simulink model "eightenPulseRectifier"  (R2024a)
settings: Solver=VariableStepAuto  StartTime=0.0  StopTime=.2  MaxStep=.0001  RelTol=1e-3
libraries: spsThyristorLib x60, spsVoltageMeasurementLib x47, spsControlledVoltageSourceLib x15, spsSeriesRLCBranchLib x9, spsZigzagPhaseShiftingTransformerLib x8, spsGroundLib x6, spsThreePhaseTransformerTwoWindingsLib x4, spsMeanLib x3, spsUniversalBridgeLib x3, slpidlib x1, simulink_extras x1, sps_lib x1
(part 1 of 2)
settings Model: Creator=User  LastModifiedBy=Admin

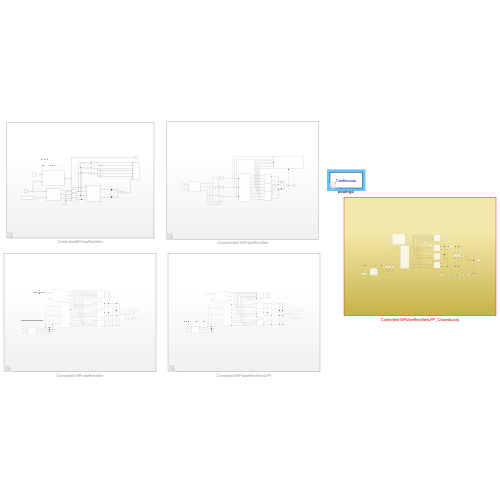
[thumbnail: Simulink's stored preview of the top-level diagram]
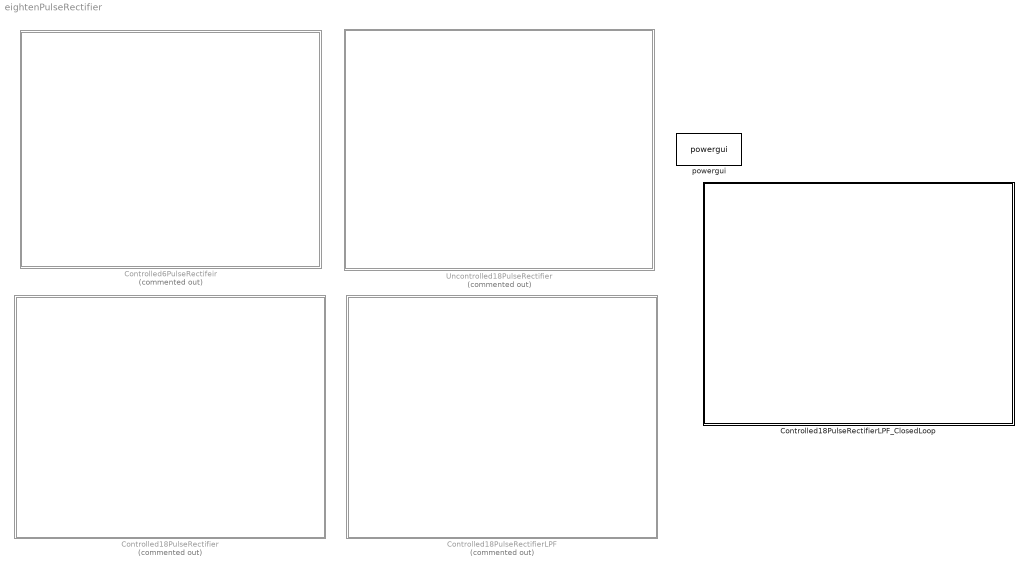
== system eightenPulseRectifier ==
  Controlled18PulseRectifier : Subsystem  Commented=on
  Controlled18PulseRectifierLPF : Subsystem  Commented=on
  Controlled18PulseRectifierLPF_ClosedLoop : Subsystem
  Controlled6PulseRectifeir : Subsystem  Commented=on
  Uncontrolled18PulseRectifier : Subsystem  Commented=on
  powergui : sps_lib/powergui  Priority=1  SimulationMode=Continuous  SampleTime=50e-6  frequency=60  Iterations=50  frequencyindice=0  Pbase=100e6  ErrMax=1e-4  UnitsV=kV  UnitsW=MW  buscounter=0  FunctionMessages=off  echomessages=off  EnableUseOfTLC=off  CurrentSourceSwitches=off  DisableSnubberDevices=off  DisableRonSwitches=off  DisableVfSwitches=off  DisplayEquations=off  AutomaticDiscreteSolvers=off  SolverType=Tustin/Backward Euler (TBE)  Interpol=off  ExternalGateDelay=off  methode=off  Ts=100  x0status=blocks  SPID=on  SwTol=0  HookPort=off  NonlinearTolerance=1e-4  nMaxIteration=100  ContinueOnMaxIteration=off  RestoreLinks=warning  ResistiveCurrentMeasurement=off  Frange=[0:2:500]  Ylog=off  Xlog=on  ShowGrid=off  save=off  variable=ZData  structure=0  ZoomFFT=off  StartTime=0.0  cycles=1  DisplayStyle=1  fundamental=60  FreqAxis=off  MaxFrequency=1000  frequencyindicesteady=1  RmsSteady=1  display=off

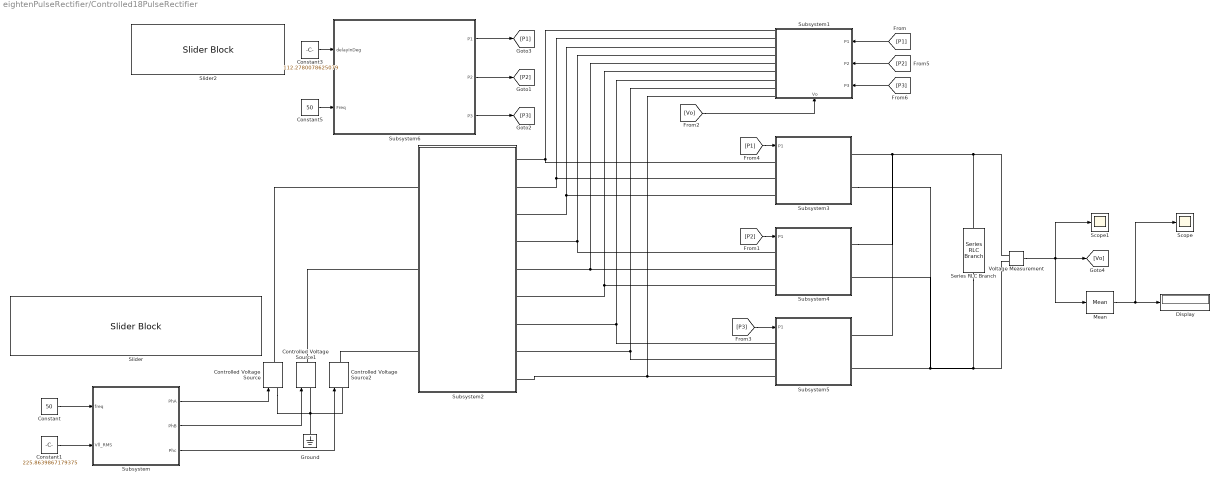
== system eightenPulseRectifier/Controlled18PulseRectifier ==
  Constant : Constant  Value=50
  Constant1 : Constant  Value=225.8639867179375
  Constant3 : Constant  Value=112.2780078625079
  Constant5 : Constant  Value=50
  Controlled Voltage Source : spsControlledVoltageSourceLib/Controlled Voltage Source  Initialize=on  Source_Type=AC  Amplitude=0  Phase=0  Frequency=0  Measurements=None
  Controlled Voltage Source1 : spsControlledVoltageSourceLib/Controlled Voltage Source  Initialize=on  Source_Type=AC  Amplitude=0  Phase=0  Frequency=0  Measurements=None
  Controlled Voltage Source2 : spsControlledVoltageSourceLib/Controlled Voltage Source  Initialize=on  Source_Type=AC  Amplitude=0  Phase=0  Frequency=0  Measurements=None
  Display : Display
  Ground : spsGroundLib/Ground  LConnTagsString=a
  Mean : spsMeanLib/Mean  Freq=60  Vinit=0  Ts=0
  Scope : Scope
  Scope1 : Scope
  Series RLC Branch : spsSeriesRLCBranchLib/Series RLC Branch  LConnTagsString=__new0  RConnTagsString=__new0  BranchType=R  Resistance=1.45  Inductance=1e-3  SetiL0=off  InitialCurrent=0  Capacitance=1e-6  Setx0=off  InitialVoltage=0  Measurements=None
  Slider : SliderBlock  ScaleMin=187  ScaleMax=253
  Slider2 : SliderBlock  ScaleMin=50  ScaleMax=180
  Subsystem : Subsystem
  Subsystem1 : Subsystem
      settings: PortSchema="{\"entries\":[{\"content\":{\"sides\":[{\"content\":{\"connectorIds\":[\"LConn1\",\"LConn2\",\"LConn3\",\"LConn4\",\"LConn5\",\"LConn6\",\"LConn7\",\"LConn8\",\"LConn9\"]},\"type\":\"ConnectorPlacement.EquallySpacedRectSide\",\"uuid\":\"c528b960-0f89-4916-bc59-feafc106a6fa\"},{\"content\":{\"connectorIds\":[\"In2\",\"In3\",\"In4\"],\"side\":\"RIGHT\"},\"type\":\"ConnectorPlacement.EquallySpacedRectSide\",\"uuid\":\"71a864a5-f7f4-48a7-95f9-d8a7d95b84d2\"},{\"content\":{\"side\":\"TOP\"},\"type\":\"ConnectorPlacement.EquallySpacedRectSide\",\"uuid\":\"57c5c08c-8233-4b40-a9fb-e09e67286da5\"},{\"content\":{\"connectorIds\":[\"In1\"],\"side\":\"BOTTOM\"},\"type\":\"ConnectorPlacement.EquallySpacedRectSide\",\"uuid\":\"030adcd8-0531-402c-81c9-62e294f4d5af\"}]},\"type\":\"ConnectorPlacement.EquallySpacedConnector\",\"uuid\":\"216ad3eb-0ca6-4d39-b862-04814928268f\"}],\"packageUris\":[\"http://schema.mathworks.com/mf0/Connector/R2020b\"],\"version\":\"1.0\"}"
  Subsystem2 : Subsystem
  Subsystem3 : Subsystem
  Subsystem4 : Subsystem
  Subsystem5 : Subsystem
  Subsystem6 : Subsystem
  Voltage Measurement : spsVoltageMeasurementLib/Voltage Measurement  PhasorSimulation=off  OutputType=Complex  PSBequivalent=0
  wires:
  Constant/1 -> Subsystem/1(freq)
  Constant1/1 -> Subsystem/2(Vll_RMS)
  Subsystem/3(Phc) -> Controlled Voltage Source2/1
  Subsystem/2(PhB) -> Controlled Voltage Source1/1
  Subsystem/1(PhA) -> Controlled Voltage Source/1
  [P3] -> Subsystem5/1(P1)
  Subsystem6/2(P2) -> [P2]
  Subsystem6/3(P3) -> [P3]
  Voltage Measurement/1 -> Mean/1, [Vo], Scope1/1
  [Vo] -> Subsystem1/1(Vo)
  [P1] -> Subsystem3/1(P1)
  [P2] -> Subsystem4/1(P1)
  Subsystem6/1(P1) -> [P1]
  [P1] -> Subsystem1/2(P1)
  [P2] -> Subsystem1/3(P2)
  [P3] -> Subsystem1/4(P3)
  Constant5/1 -> Subsystem6/2(Freq)
  Constant3/1 -> Subsystem6/1(delayInDeg)
  Mean/1 -> Scope/1, Display/1
  connections:
  Subsystem1/LConn9 -- Subsystem2/RConn9 -- Subsystem5/LConn3
  Subsystem1/LConn6 -- Subsystem4/LConn3 -- Subsystem2/RConn6
  Controlled Voltage Source/RConn1 -- Subsystem2/LConn1
  Subsystem1/LConn5 -- Subsystem2/RConn5 -- Subsystem4/LConn2
  Subsystem1/LConn7 -- Subsystem5/LConn1 -- Subsystem2/RConn7
  Subsystem1/LConn3 -- Subsystem2/RConn3 -- Subsystem3/LConn3
  Ground/LConn1 -- Controlled Voltage Source/LConn1 -- Controlled Voltage Source1/LConn1 -- Controlled Voltage Source2/LConn1
  Subsystem3/LConn2 -- Subsystem1/LConn2 -- Subsystem2/RConn2
  Voltage Measurement/LConn1 -- Subsystem4/RConn1 -- Subsystem5/RConn1 -- Subsystem3/RConn1 -- Series RLC Branch/LConn1
  Series RLC Branch/RConn1 -- Subsystem3/RConn2 -- Subsystem4/RConn2 -- Subsystem5/RConn2 -- Voltage Measurement/LConn2
  Subsystem1/LConn8 -- Subsystem5/LConn2 -- Subsystem2/RConn8
  Subsystem1/LConn4 -- Subsystem4/LConn1 -- Subsystem2/RConn4
  Controlled Voltage Source2/RConn1 -- Subsystem2/LConn3
  Controlled Voltage Source1/RConn1 -- Subsystem2/LConn2
  Subsystem1/LConn1 -- Subsystem3/LConn1 -- Subsystem2/RConn1

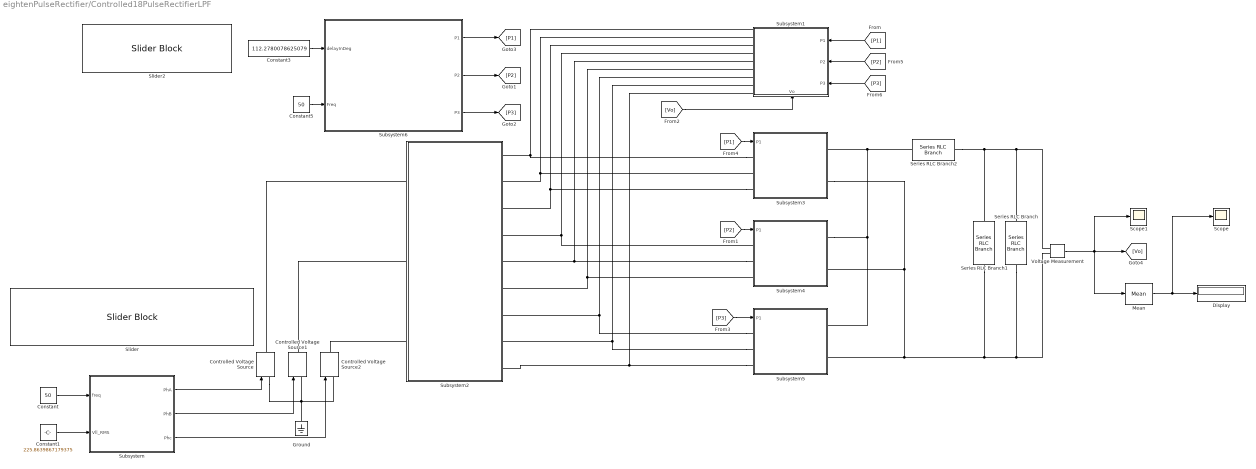
== system eightenPulseRectifier/Controlled18PulseRectifierLPF ==
  Constant : Constant  Value=50
  Constant1 : Constant  Value=225.8639867179375
  Constant3 : Constant  Value=112.2780078625079
  Constant5 : Constant  Value=50
  Controlled Voltage Source : spsControlledVoltageSourceLib/Controlled Voltage Source  Initialize=on  Source_Type=AC  Amplitude=0  Phase=0  Frequency=0  Measurements=None
  Controlled Voltage Source1 : spsControlledVoltageSourceLib/Controlled Voltage Source  Initialize=on  Source_Type=AC  Amplitude=0  Phase=0  Frequency=0  Measurements=None
  Controlled Voltage Source2 : spsControlledVoltageSourceLib/Controlled Voltage Source  Initialize=on  Source_Type=AC  Amplitude=0  Phase=0  Frequency=0  Measurements=None
  Display : Display
  Ground : spsGroundLib/Ground  LConnTagsString=a
  Mean : spsMeanLib/Mean  Freq=60  Vinit=0  Ts=0
  Scope : Scope
  Scope1 : Scope
  Series RLC Branch : spsSeriesRLCBranchLib/Series RLC Branch  LConnTagsString=__new0  RConnTagsString=__new0  BranchType=R  Resistance=1.45  Inductance=1e-3  SetiL0=off  InitialCurrent=0  Capacitance=1e-6  Setx0=off  InitialVoltage=0  Measurements=None
  Series RLC Branch1 : spsSeriesRLCBranchLib/Series RLC Branch  LConnTagsString=__new0  RConnTagsString=__new0  BranchType=C  Resistance=1.45  Inductance=1e-3  SetiL0=off  InitialCurrent=0  Capacitance=1500e-6  Setx0=off  InitialVoltage=0  Measurements=None
  Series RLC Branch2 : spsSeriesRLCBranchLib/Series RLC Branch  LConnTagsString=__new0  RConnTagsString=__new0  BranchType=L  Resistance=1.45  Inductance=2e-3  SetiL0=off  InitialCurrent=0  Capacitance=1e-6  Setx0=off  InitialVoltage=0  Measurements=None
  Slider : SliderBlock  ScaleMin=187  ScaleMax=253
  Slider2 : SliderBlock  ScaleMin=50  ScaleMax=180
  Subsystem : Subsystem
  Subsystem1 : Subsystem
      settings: PortSchema="{\"entries\":[{\"content\":{\"sides\":[{\"content\":{\"connectorIds\":[\"LConn1\",\"LConn2\",\"LConn3\",\"LConn4\",\"LConn5\",\"LConn6\",\"LConn7\",\"LConn8\",\"LConn9\"]},\"type\":\"ConnectorPlacement.EquallySpacedRectSide\",\"uuid\":\"c528b960-0f89-4916-bc59-feafc106a6fa\"},{\"content\":{\"connectorIds\":[\"In2\",\"In3\",\"In4\"],\"side\":\"RIGHT\"},\"type\":\"ConnectorPlacement.EquallySpacedRectSide\",\"uuid\":\"71a864a5-f7f4-48a7-95f9-d8a7d95b84d2\"},{\"content\":{\"side\":\"TOP\"},\"type\":\"ConnectorPlacement.EquallySpacedRectSide\",\"uuid\":\"57c5c08c-8233-4b40-a9fb-e09e67286da5\"},{\"content\":{\"connectorIds\":[\"In1\"],\"side\":\"BOTTOM\"},\"type\":\"ConnectorPlacement.EquallySpacedRectSide\",\"uuid\":\"030adcd8-0531-402c-81c9-62e294f4d5af\"}]},\"type\":\"ConnectorPlacement.EquallySpacedConnector\",\"uuid\":\"216ad3eb-0ca6-4d39-b862-04814928268f\"}],\"packageUris\":[\"http://schema.mathworks.com/mf0/Connector/R2020b\"],\"version\":\"1.0\"}"
  Subsystem2 : Subsystem
  Subsystem3 : Subsystem
  Subsystem4 : Subsystem
  Subsystem5 : Subsystem
  Subsystem6 : Subsystem
  Voltage Measurement : spsVoltageMeasurementLib/Voltage Measurement  PhasorSimulation=off  OutputType=Complex  PSBequivalent=0
  wires:
  Mean/1 -> Display/1, Scope/1
  Constant3/1 -> Subsystem6/1(delayInDeg)
  Constant5/1 -> Subsystem6/2(Freq)
  [P3] -> Subsystem1/4(P3)
  [P2] -> Subsystem1/3(P2)
  [P1] -> Subsystem1/2(P1)
  Subsystem6/1(P1) -> [P1]
  [P2] -> Subsystem4/1(P1)
  [P1] -> Subsystem3/1(P1)
  [Vo] -> Subsystem1/1(Vo)
  Voltage Measurement/1 -> Scope1/1, [Vo], Mean/1
  Subsystem6/3(P3) -> [P3]
  Subsystem6/2(P2) -> [P2]
  [P3] -> Subsystem5/1(P1)
  Subsystem/1(PhA) -> Controlled Voltage Source/1
  Subsystem/2(PhB) -> Controlled Voltage Source1/1
  Subsystem/3(Phc) -> Controlled Voltage Source2/1
  Constant1/1 -> Subsystem/2(Vll_RMS)
  Constant/1 -> Subsystem/1(freq)
  connections:
  Subsystem3/LConn1 -- Subsystem2/RConn1 -- Subsystem1/LConn1
  Controlled Voltage Source1/RConn1 -- Subsystem2/LConn2
  Controlled Voltage Source2/RConn1 -- Subsystem2/LConn3
  Subsystem2/RConn4 -- Subsystem1/LConn4 -- Subsystem4/LConn1
  Subsystem5/LConn2 -- Subsystem2/RConn8 -- Subsystem1/LConn8
  Voltage Measurement/LConn2 -- Series RLC Branch1/RConn1 -- Subsystem5/RConn2 -- Subsystem3/RConn2 -- Subsystem4/RConn2 -- Series RLC Branch/RConn1
  Subsystem3/RConn1 -- Series RLC Branch2/LConn1 -- Subsystem5/RConn1 -- Subsystem4/RConn1
  Subsystem2/RConn2 -- Subsystem1/LConn2 -- Subsystem3/LConn2
  Controlled Voltage Source2/LConn1 -- Controlled Voltage Source1/LConn1 -- Controlled Voltage Source/LConn1 -- Ground/LConn1
  Subsystem3/LConn3 -- Subsystem2/RConn3 -- Subsystem1/LConn3
  Subsystem5/LConn1 -- Subsystem2/RConn7 -- Subsystem1/LConn7
  Subsystem4/LConn2 -- Subsystem2/RConn5 -- Subsystem1/LConn5
  Controlled Voltage Source/RConn1 -- Subsystem2/LConn1
  Subsystem2/RConn6 -- Subsystem4/LConn3 -- Subsystem1/LConn6
  Subsystem5/LConn3 -- Subsystem2/RConn9 -- Subsystem1/LConn9
  Series RLC Branch/LConn1 -- Series RLC Branch1/LConn1 -- Series RLC Branch2/RConn1 -- Voltage Measurement/LConn1

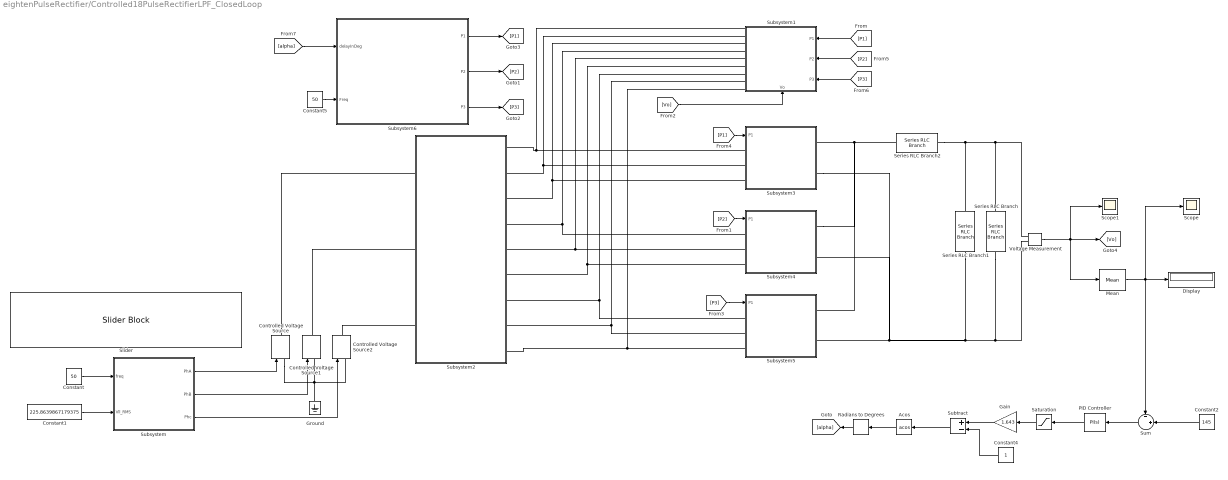
== system eightenPulseRectifier/Controlled18PulseRectifierLPF_ClosedLoop ==
  Acos : Trigonometry  Operator=acos
  Constant : Constant  Value=50
  Constant1 : Constant  Value=225.8639867179375
  Constant2 : Constant  Value=145
  Constant4 : Constant
  Constant5 : Constant  Value=50
  Controlled Voltage Source : spsControlledVoltageSourceLib/Controlled Voltage Source  Initialize=on  Source_Type=AC  Amplitude=0  Phase=0  Frequency=0  Measurements=None
  Controlled Voltage Source1 : spsControlledVoltageSourceLib/Controlled Voltage Source  Initialize=on  Source_Type=AC  Amplitude=0  Phase=0  Frequency=0  Measurements=None
  Controlled Voltage Source2 : spsControlledVoltageSourceLib/Controlled Voltage Source  Initialize=on  Source_Type=AC  Amplitude=0  Phase=0  Frequency=0  Measurements=None
  Display : Display
  Gain : Gain  Gain=1.643
  Ground : spsGroundLib/Ground  LConnTagsString=a
  Mean : spsMeanLib/Mean  Freq=60  Vinit=0  Ts=0
  PID Controller : slpidlib/PID Controller  Controller=PI  Form=Parallel  TimeDomain=Continuous-time  UseExternalTs=off  SampleTime=-1  IntegratorMethod=Forward Euler  FilterMethod=Forward Euler  ControllerParametersSource=internal  P=.02  I=5  UseKiTs=off  D=0  UseExternalDerivativeSource=off  N=100  UseFilter=on  TunerSelectOption=Transfer Function Based (PID Tuner App)  InitialConditionSource=internal  InitialConditionForIntegrator=0  InitialConditionForFilter=0  DifferentiatorICPrevScaledInput=0  ExternalReset=none  TrackingMode=off  Kt=1  LimitOutput=off  SatLimitsSource=internal  UpperSaturationLimit=.95  LowerSaturationLimit=.1  LinearizeAsGain=on  AntiWindupMode=clamping  Kb=1  LimitIntegrator=off  UpperIntegratorSaturationLimit=inf  LowerIntegratorSaturationLimit=-inf  POutMin=[]  POutMax=[]  IOutMin=[]  IOutMax=[]  DOutMin=[]  DOutMax=[]  NOutMin=[]  NOutMax=[]  SumOutMin=[]  SumOutMax=[]  SaturationOutMin=[]  SaturationOutMax=[]  PParamMin=[]  PParamMax=[]  IParamMin=[]  IParamMax=[]  DParamMin=[]  DParamMax=[]  NParamMin=[]  NParamMax=[]  KbParamMin=[]  KbParamMax=[]  KtParamMin=[]  KtParamMax=[]  KbOutMin=[]  KbOutMax=[]  KtOutMin=[]  KtOutMax=[]  IntegratorOutMin=[]  IntegratorOutMax=[]  FilterOutMin=[]  FilterOutMax=[]  SumI1OutMin=[]  SumI1OutMax=[]  SumI2OutMin=[]  SumI2OutMax=[]  SumI3OutMin=[]  SumI3OutMax=[]  SumI4OutMin=[]  SumI4OutMax=[]  SumDOutMin=[]  SumDOutMax=[]  DifferentiatorOutMin=[]  DifferentiatorOutMax=[]  FilterDiffOutCoefMin=[]  FilterDiffOutCoefMax=[]  ReciprocalOutMin=[]  ReciprocalOutMax=[]  SumDenOutMin=[]  SumDenOutMax=[]  SumNumOutMin=[]  SumNumOutMax=[]  DivideOutMin=[]  DivideOutMax=[]  UdiffTsProdOutMin=[]  UdiffTsProdOutMax=[]  NTsProdOutMin=[]  NTsProdOutMax=[]  UintegralTsProdOutMin=[]  UintegralTsProdOutMax=[]  UngainTsProdOutMin=[]  UngainTsProdOutMax=[]  ClampingZeroOutDataTypeStr=Inherit: Inherit via back propagation  ClampingZeroOutMin=[]  ClampingZeroOutMax=[]  FilterDenConstantOutDataTypeStr=Inherit: Inherit via back propagation  FilterDenConstantOutMin=[]  FilterDenConstantOutMax=[]  PCopyOutDataTypeStr=Inherit: Inherit via back propagation  PCopyOutMin=[]  PCopyOutMax=[]  NCopyOutDataTypeStr=Inherit: Inherit via back propagation  NCopyOutMin=[]  NCopyOutMax=[]  IntegratorContinuousStateAttributes=''  IntegratorStateMustResolveToSignalObject=off  IntegratorRTWStateStorageClass=Auto  FilterContinuousStateAttributes=''  FilterStateMustResolveToSignalObject=off  FilterRTWStateStorageClass=Auto  ParallelPVariant=InternalParameters  IdealPVariant=Disabled  IVariant=InternalParameters  DVariant=Disabled  IntegratorVariant=Continuous  SatVariant=Disabled  AWVariant=Passthrough  PCopyVariant=Disabled  TRVariant=Disabled  FdbkBlocksVariant=Forward  IdealPFdbkVariant=Disabled  SatFdbkVariant=Disabled  DerivativeFilterVariant=Disabled  NVariant=Disabled  NCopyVariant=Disabled_SignalSpec  FilterICVariant=Disabled  IntegratorICVariant=InternalICs  ExternalResetVariant=Disabled  TRSumVariant=Passthrough  SumFdbkVariant=Disabled  SumVariant=Sum_PI  TsampFilterVariant=InternalTs  TsampNgainVariant=Passthrough  TsampIntegralVariant=Disabled_SignalSpec  ExternalSaturationOutDataTypeStr=Inherit: Same as second input  DerivativeSourceVariant=Disabled
  Radians to Degrees : simulink_extras/Transformations/Radians to Degrees
  Saturation : Saturate  UpperLimit=.95  LowerLimit=.1
  Scope : Scope
  Scope1 : Scope
  Series RLC Branch : spsSeriesRLCBranchLib/Series RLC Branch  LConnTagsString=__new0  RConnTagsString=__new0  BranchType=R  Resistance=1.45  Inductance=1e-3  SetiL0=off  InitialCurrent=0  Capacitance=1e-6  Setx0=off  InitialVoltage=0  Measurements=None
  Series RLC Branch1 : spsSeriesRLCBranchLib/Series RLC Branch  LConnTagsString=__new0  RConnTagsString=__new0  BranchType=C  Resistance=1.45  Inductance=1e-3  SetiL0=off  InitialCurrent=0  Capacitance=1500e-6  Setx0=off  InitialVoltage=0  Measurements=None
  Series RLC Branch2 : spsSeriesRLCBranchLib/Series RLC Branch  LConnTagsString=__new0  RConnTagsString=__new0  BranchType=L  Resistance=1.45  Inductance=2e-3  SetiL0=off  InitialCurrent=0  Capacitance=1e-6  Setx0=off  InitialVoltage=0  Measurements=None
  Slider : SliderBlock  ScaleMin=187  ScaleMax=253
  Subsystem : Subsystem
  Subsystem1 : Subsystem
      settings: PortSchema="{\"entries\":[{\"content\":{\"sides\":[{\"content\":{\"connectorIds\":[\"LConn1\",\"LConn2\",\"LConn3\",\"LConn4\",\"LConn5\",\"LConn6\",\"LConn7\",\"LConn8\",\"LConn9\"]},\"type\":\"ConnectorPlacement.EquallySpacedRectSide\",\"uuid\":\"c528b960-0f89-4916-bc59-feafc106a6fa\"},{\"content\":{\"connectorIds\":[\"In2\",\"In3\",\"In4\"],\"side\":\"RIGHT\"},\"type\":\"ConnectorPlacement.EquallySpacedRectSide\",\"uuid\":\"71a864a5-f7f4-48a7-95f9-d8a7d95b84d2\"},{\"content\":{\"side\":\"TOP\"},\"type\":\"ConnectorPlacement.EquallySpacedRectSide\",\"uuid\":\"57c5c08c-8233-4b40-a9fb-e09e67286da5\"},{\"content\":{\"connectorIds\":[\"In1\"],\"side\":\"BOTTOM\"},\"type\":\"ConnectorPlacement.EquallySpacedRectSide\",\"uuid\":\"030adcd8-0531-402c-81c9-62e294f4d5af\"}]},\"type\":\"ConnectorPlacement.EquallySpacedConnector\",\"uuid\":\"216ad3eb-0ca6-4d39-b862-04814928268f\"}],\"packageUris\":[\"http://schema.mathworks.com/mf0/Connector/R2020b\"],\"version\":\"1.0\"}"
  Subsystem2 : Subsystem
  Subsystem3 : Subsystem
  Subsystem4 : Subsystem
  Subsystem5 : Subsystem
  Subsystem6 : Subsystem
  Subtract : Sum  Inputs=+-
  Sum : Sum  Inputs=-|+||
  Voltage Measurement : spsVoltageMeasurementLib/Voltage Measurement  PhasorSimulation=off  OutputType=Complex  PSBequivalent=0
  wires:
  Constant/1 -> Subsystem/1(freq)
  Constant1/1 -> Subsystem/2(Vll_RMS)
  Subsystem/3(Phc) -> Controlled Voltage Source2/1
  Subsystem/2(PhB) -> Controlled Voltage Source1/1
  Subsystem/1(PhA) -> Controlled Voltage Source/1
  [P3] -> Subsystem5/1(P1)
  Subsystem6/2(P2) -> [P2]
  Subsystem6/3(P3) -> [P3]
  Voltage Measurement/1 -> Mean/1, [Vo], Scope1/1
  [Vo] -> Subsystem1/1(Vo)
  [P1] -> Subsystem3/1(P1)
  [P2] -> Subsystem4/1(P1)
  Subsystem6/1(P1) -> [P1]
  [P1] -> Subsystem1/2(P1)
  [P2] -> Subsystem1/3(P2)
  [P3] -> Subsystem1/4(P3)
  Constant5/1 -> Subsystem6/2(Freq)
  Mean/1 -> Display/1, Sum/1, Scope/1
  Sum/1 -> PID Controller/1
  Constant2/1 -> Sum/2
  PID Controller/1 -> Saturation/1
  Subtract/1 -> Acos/1
  Acos/1 -> Radians to Degrees/1
  Radians to Degrees/1 -> [alpha]
  [alpha] -> Subsystem6/1(delayInDeg)
  Saturation/1 -> Gain/1
  Gain/1 -> Subtract/1
  Constant4/1 -> Subtract/2
  connections:
  Series RLC Branch1/LConn1 -- Series RLC Branch2/RConn1 -- Voltage Measurement/LConn1 -- Series RLC Branch/LConn1
  Subsystem1/LConn9 -- Subsystem2/RConn9 -- Subsystem5/LConn3
  Subsystem1/LConn6 -- Subsystem4/LConn3 -- Subsystem2/RConn6
  Controlled Voltage Source/RConn1 -- Subsystem2/LConn1
  Subsystem1/LConn5 -- Subsystem2/RConn5 -- Subsystem4/LConn2
  Subsystem1/LConn7 -- Subsystem2/RConn7 -- Subsystem5/LConn1
  Subsystem1/LConn3 -- Subsystem2/RConn3 -- Subsystem3/LConn3
  Ground/LConn1 -- Controlled Voltage Source/LConn1 -- Controlled Voltage Source1/LConn1 -- Controlled Voltage Source2/LConn1
  Subsystem3/LConn2 -- Subsystem1/LConn2 -- Subsystem2/RConn2
  Series RLC Branch2/LConn1 -- Subsystem4/RConn1 -- Subsystem5/RConn1 -- Subsystem3/RConn1
  Series RLC Branch1/RConn1 -- Subsystem4/RConn2 -- Subsystem3/RConn2 -- Subsystem5/RConn2 -- Series RLC Branch/RConn1 -- Voltage Measurement/LConn2
  Subsystem1/LConn8 -- Subsystem2/RConn8 -- Subsystem5/LConn2
  Subsystem4/LConn1 -- Subsystem1/LConn4 -- Subsystem2/RConn4
  Controlled Voltage Source2/RConn1 -- Subsystem2/LConn3
  Controlled Voltage Source1/RConn1 -- Subsystem2/LConn2
  Subsystem1/LConn1 -- Subsystem2/RConn1 -- Subsystem3/LConn1

== system eightenPulseRectifier/Controlled6PulseRectifeir ==
  Constant : Constant  Value=50
  Constant1 : Constant  Value=225.8639867179375
  Constant2 : Constant  Value=30
  Controlled Voltage Source : spsControlledVoltageSourceLib/Controlled Voltage Source  Initialize=on  Source_Type=AC  Amplitude=0  Phase=0  Frequency=0  Measurements=None
  Controlled Voltage Source1 : spsControlledVoltageSourceLib/Controlled Voltage Source  Initialize=on  Source_Type=AC  Amplitude=0  Phase=0  Frequency=0  Measurements=None
  Controlled Voltage Source2 : spsControlledVoltageSourceLib/Controlled Voltage Source  Initialize=on  Source_Type=AC  Amplitude=0  Phase=0  Frequency=0  Measurements=None
  Gain : Gain  Gain=-1
  Gain1 : Gain  Gain=-1
  Gain2 : Gain  Gain=-1
  Ground : spsGroundLib/Ground  LConnTagsString=a
  Scope : Scope  NumInputPorts=7
  Scope1 : Scope
  Series RLC Branch : spsSeriesRLCBranchLib/Series RLC Branch  LConnTagsString=__new0  RConnTagsString=__new0  BranchType=R  Resistance=10000  Inductance=1e-3  SetiL0=off  InitialCurrent=0  Capacitance=1e-6  Setx0=off  InitialVoltage=0  Measurements=None
  Slider : SliderBlock  ScaleMin=30  ScaleMax=180
  Subsystem : Subsystem
  Subsystem4 : Subsystem
  Subsystem5 : Subsystem
  Voltage Measurement{,1..3} (4 alike) : spsVoltageMeasurementLib/Voltage Measurement  PhasorSimulation=off  OutputType=Complex  PSBequivalent=0
  wires:
  Voltage Measurement1/1 -> Gain1/1, Scope/3  "Vbc"
  Constant/1 -> Subsystem/2(Freq), Subsystem5/1(freq)
  Gain/1 -> Scope/2  "Vba"
  Voltage Measurement2/1 -> Gain2/1, Scope/5  "Vca"
  Voltage Measurement/1 -> Gain/1, Scope/1  "Vab"
  Subsystem5/1(PhA) -> Controlled Voltage Source/1
  Voltage Measurement3/1 -> Scope/7  "Vo"
  Gain2/1 -> Scope/6  "Vac"
  Gain1/1 -> Scope/4  "Vcb"
  Subsystem5/3(Phc) -> Controlled Voltage Source2/1
  Constant1/1 -> Subsystem5/2(Vll_RMS)
  Subsystem5/2(PhB) -> Controlled Voltage Source1/1
  Constant2/1 -> Subsystem/1(delayInDeg)
  Subsystem/1(P1) -> Subsystem4/1(P1), Scope1/1
  connections:
  Controlled Voltage Source/RConn1 -- Voltage Measurement/LConn1 -- Voltage Measurement2/LConn2 -- Subsystem4/LConn1
  Controlled Voltage Source1/RConn1 -- Voltage Measurement/LConn2 -- Voltage Measurement1/LConn1 -- Subsystem4/LConn2
  Controlled Voltage Source2/LConn1 -- Ground/LConn1 -- Controlled Voltage Source/LConn1 -- Controlled Voltage Source1/LConn1
  Controlled Voltage Source2/RConn1 -- Voltage Measurement1/LConn2 -- Voltage Measurement2/LConn1 -- Subsystem4/LConn3
  Series RLC Branch/LConn1 -- Voltage Measurement3/LConn1 -- Subsystem4/RConn1
  Series RLC Branch/RConn1 -- Voltage Measurement3/LConn2 -- Subsystem4/RConn2

== system eightenPulseRectifier/Uncontrolled18PulseRectifier ==
  Constant : Constant  Value=50
  Constant1 : Constant  Value=200
  Controlled Voltage Source : spsControlledVoltageSourceLib/Controlled Voltage Source  Initialize=on  Source_Type=AC  Amplitude=0  Phase=0  Frequency=0  Measurements=None
  Controlled Voltage Source1 : spsControlledVoltageSourceLib/Controlled Voltage Source  Initialize=on  Source_Type=AC  Amplitude=0  Phase=0  Frequency=0  Measurements=None
  Controlled Voltage Source2 : spsControlledVoltageSourceLib/Controlled Voltage Source  Initialize=on  Source_Type=AC  Amplitude=0  Phase=0  Frequency=0  Measurements=None
  Ground : spsGroundLib/Ground  LConnTagsString=a
  Scope : Scope  NumInputPorts=3
  Scope1 : Scope
  Series RLC Branch : spsSeriesRLCBranchLib/Series RLC Branch  LConnTagsString=__new0  RConnTagsString=__new0  BranchType=R  Resistance=2000  Inductance=1e-3  SetiL0=off  InitialCurrent=0  Capacitance=1e-6  Setx0=off  InitialVoltage=0  Measurements=None
  Subsystem : Subsystem
  Subsystem1 : Subsystem
      settings: PortSchema="{\"entries\":[{\"content\":{\"sides\":[{\"content\":{\"connectorIds\":[\"LConn1\",\"LConn2\",\"LConn3\",\"LConn4\",\"LConn5\",\"LConn6\",\"LConn7\",\"LConn8\",\"LConn9\"]},\"type\":\"ConnectorPlacement.EquallySpacedRectSide\",\"uuid\":\"c528b960-0f89-4916-bc59-feafc106a6fa\"},{\"content\":{\"side\":\"RIGHT\"},\"type\":\"ConnectorPlacement.EquallySpacedRectSide\",\"uuid\":\"71a864a5-f7f4-48a7-95f9-d8a7d95b84d2\"},{\"content\":{\"side\":\"TOP\"},\"type\":\"ConnectorPlacement.EquallySpacedRectSide\",\"uuid\":\"57c5c08c-8233-4b40-a9fb-e09e67286da5\"},{\"content\":{\"connectorIds\":[\"In1\"],\"side\":\"BOTTOM\"},\"type\":\"ConnectorPlacement.EquallySpacedRectSide\",\"uuid\":\"f6f9f7ac-8837-43ce-91db-f6801ff1a468\"}]},\"type\":\"ConnectorPlacement.EquallySpacedConnector\",\"uuid\":\"216ad3eb-0ca6-4d39-b862-04814928268f\"}],\"packageUris\":[\"http://schema.mathworks.com/mf0/Connector/R2020b\"],\"version\":\"1.0\"}"
  Subsystem2 : Subsystem
  Universal Bridge1 : spsUniversalBridgeLib/Universal Bridge  Arms=3  SnubberResistance=1e5  SnubberCapacitance=inf  Device=Diodes  Ron=1e-3  Lon=0  ForwardVoltages="[  0  0  ]"  ForwardVoltage=0  GTOparameters=[ 10e-6 , 20e-6 ]  IGBTparameters=[ 1e-6 , 2e-6 ]  Measurements=None  Measurements_2=None  converterType=Rectifier
  Universal Bridge2 : spsUniversalBridgeLib/Universal Bridge  Arms=3  SnubberResistance=1e5  SnubberCapacitance=inf  Device=Diodes  Ron=1e-3  Lon=0  ForwardVoltages="[  0  0  ]"  ForwardVoltage=0  GTOparameters=[ 10e-6 , 20e-6 ]  IGBTparameters=[ 1e-6 , 2e-6 ]  Measurements=None  Measurements_2=None  converterType=Rectifier
  Universal Bridge3 : spsUniversalBridgeLib/Universal Bridge  Arms=3  SnubberResistance=1e5  SnubberCapacitance=inf  Device=Diodes  Ron=1e-3  Lon=0  ForwardVoltages="[  0  0  ]"  ForwardVoltage=0  GTOparameters=[ 10e-6 , 20e-6 ]  IGBTparameters=[ 1e-6 , 2e-6 ]  Measurements=None  Measurements_2=None  converterType=Rectifier
  Voltage Measurement : spsVoltageMeasurementLib/Voltage Measurement  PhasorSimulation=off  OutputType=Complex  PSBequivalent=0
  wires:
  Subsystem/1(PhA) -> Controlled Voltage Source/1, Scope/1
  Subsystem/2(PhB) -> Scope/2, Controlled Voltage Source1/1
  Subsystem/3(Phc) -> Scope/3, Controlled Voltage Source2/1
  Constant1/1 -> Subsystem/2(Vll_RMS)
  Constant/1 -> Subsystem/1(freq)
  Voltage Measurement/1 -> Scope1/1, Subsystem1/1(" ")
  connections:
  Subsystem2/RConn3 -- Universal Bridge3/LConn3
  Subsystem2/RConn2 -- Universal Bridge3/LConn2
  Subsystem2/RConn1 -- Universal Bridge3/LConn1
  Subsystem2/RConn7 -- Subsystem1/LConn7 -- Universal Bridge2/LConn1
  Subsystem1/LConn2 -- Subsystem2/LConn2 -- Controlled Voltage Source1/RConn1
  Subsystem2/RConn9 -- Subsystem1/LConn9 -- Universal Bridge2/LConn3
  Subsystem2/RConn6 -- Universal Bridge1/LConn3 -- Subsystem1/LConn6
  Subsystem2/LConn1 -- Controlled Voltage Source/RConn1 -- Subsystem1/LConn1
  Subsystem2/LConn3 -- Controlled Voltage Source2/RConn1 -- Subsystem1/LConn3
  Subsystem2/RConn8 -- Subsystem1/LConn8 -- Universal Bridge2/LConn2
  Subsystem2/RConn4 -- Universal Bridge1/LConn1 -- Subsystem1/LConn4
  Controlled Voltage Source1/LConn1 -- Controlled Voltage Source2/LConn1 -- Ground/LConn1 -- Controlled Voltage Source/LConn1
  Subsystem2/RConn5 -- Universal Bridge1/LConn2 -- Subsystem1/LConn5
  Voltage Measurement/LConn1 -- Series RLC Branch/LConn1 -- Universal Bridge2/RConn1 -- Universal Bridge1/RConn1 -- Universal Bridge3/RConn1
  Voltage Measurement/LConn2 -- Series RLC Branch/RConn1 -- Universal Bridge2/RConn2 -- Universal Bridge1/RConn2 -- Universal Bridge3/RConn2

== system eightenPulseRectifier/Controlled18PulseRectifier/Subsystem ==
  freq : Inport
  Vll_RMS : Inport  Port=2
  Add : Sum
  Add1 : Sum
  Add2 : Sum
  Constant : Constant
  Gain : Gain  Gain=2*pi
  Gain1 : Gain  Gain=sqrt(2/3)
  Integrator : Integrator
  Product{,1..3} (4 alike) : Product
  Sin : Trigonometry
  Sin1 : Trigonometry
  Sin2 : Trigonometry
  phase : Constant  Value=0
  phase B : Constant  Value=-2*pi/3
  phase B1 : Constant  Value=2*pi/3
  PhA : Outport
  PhB : Outport  Port=2
  Phc : Outport  Port=3
  wires:
  Sin/1 -> Product/1
  Product3/1 -> Phc/1
  freq/1 -> Product2/1
  Product/1 -> PhA/1
  phase B1/1 -> Add2/2
  Add2/1 -> Sin2/1
  Add1/1 -> Sin1/1
  Add/1 -> Sin/1
  phase B/1 -> Add1/2
  phase/1 -> Add/2
  Vll_RMS/1 -> Gain1/1
  Constant/1 -> Integrator/1
  Integrator/1 -> Gain/1
  Product2/1 -> Add/1, Add1/1, Add2/1
  Product1/1 -> PhB/1
  Sin2/1 -> Product3/1
  Sin1/1 -> Product1/1
  Gain/1 -> Product2/2  "2pit"
  Gain1/1 -> Product1/2, Product3/2, Product/2

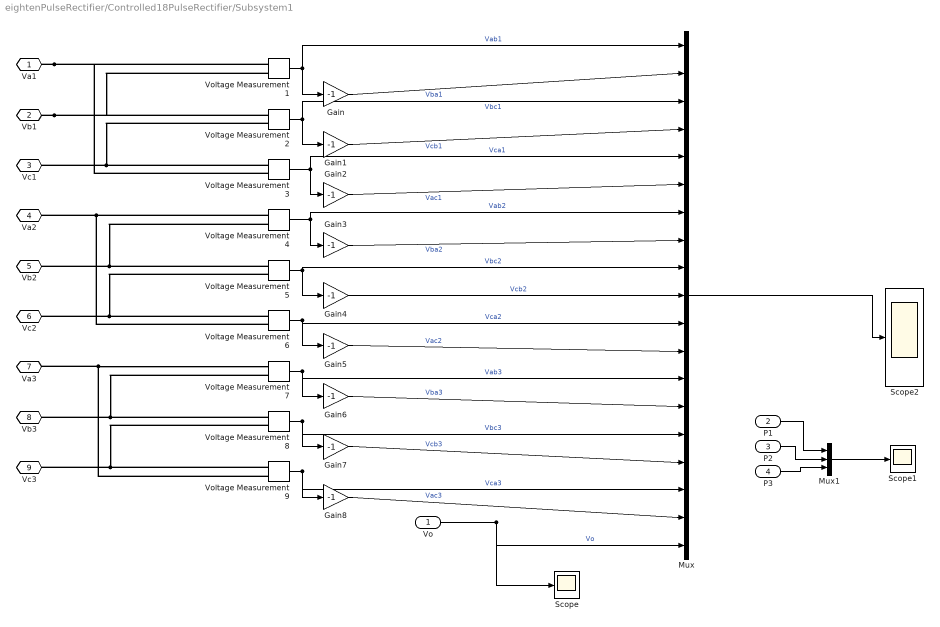
== system eightenPulseRectifier/Controlled18PulseRectifier/Subsystem1 ==
  Vo : Inport
  P1 : Inport  Port=2
  P2 : Inport  Port=3
  P3 : Inport  Port=4
  Gain{,1..8} (9 alike) : Gain  Gain=-1
  Mux : Mux  Inputs=19
  Mux1 : Mux  Inputs=3
  Scope : Scope
  Scope1 : Scope
  Scope2 : Scope
  Voltage Measurement{1..9} (9 alike) : spsVoltageMeasurementLib/Voltage Measurement  PhasorSimulation=off  OutputType=Complex  PSBequivalent=0
  Va1 : PMIOPort  Side=Left
  Vb1 : PMIOPort  Port=2  Side=Left
  Vc1 : PMIOPort  Port=3  Side=Left
  Va2 : PMIOPort  Port=4  Side=Left
  Vb2 : PMIOPort  Port=5  Side=Left
  Vc2 : PMIOPort  Port=6  Side=Left
  Va3 : PMIOPort  Port=7  Side=Left
  Vb3 : PMIOPort  Port=8  Side=Left
  Vc3 : PMIOPort  Port=9  Side=Left
  wires:
  Voltage Measurement2/1 -> Gain1/1, Mux/3  "Vbc1"
  Voltage Measurement4/1 -> Gain3/1, Mux/7  "Vab2"
  Voltage Measurement5/1 -> Gain4/1, Mux/9  "Vbc2"
  Voltage Measurement3/1 -> Gain2/1, Mux/5  "Vca1"
  Gain1/1 -> Mux/4  "Vcb1"
  Gain8/1 -> Mux/18  "Vac3"
  Gain7/1 -> Mux/16  "Vcb3"
  Voltage Measurement9/1 -> Mux/17, Gain8/1  "Vca3"
  Gain5/1 -> Mux/12  "Vac2"
  Voltage Measurement7/1 -> Gain6/1, Mux/13  "Vab3"
  Voltage Measurement6/1 -> Gain5/1, Mux/11  "Vca2"
  Voltage Measurement1/1 -> Gain/1, Mux/1  "Vab1"
  Voltage Measurement8/1 -> Mux/15, Gain7/1  "Vbc3"
  Gain4/1 -> Mux/10  "Vcb2"
  Gain2/1 -> Mux/6  "Vac1"
  Gain/1 -> Mux/2  "Vba1"
  Gain6/1 -> Mux/14  "Vba3"
  Gain3/1 -> Mux/8  "Vba2"
  Vo/1 -> Scope/1, Mux/19  "Vo"
  Mux/1 -> Scope2/1
  P1/1 -> Mux1/1
  P2/1 -> Mux1/2
  P3/1 -> Mux1/3
  Mux1/1 -> Scope1/1
  connections:
  Voltage Measurement6/LConn1 -- Voltage Measurement5/LConn2 -- Vc2/RConn1
  Voltage Measurement9/LConn1 -- Voltage Measurement8/LConn2 -- Vc3/RConn1
  Voltage Measurement5/LConn1 -- Voltage Measurement4/LConn2 -- Vb2/RConn1
  Va1/RConn1 -- Voltage Measurement1/LConn1 -- Voltage Measurement3/LConn2
  Voltage Measurement4/LConn1 -- Voltage Measurement6/LConn2 -- Va2/RConn1
  Voltage Measurement9/LConn2 -- Va3/RConn1 -- Voltage Measurement7/LConn1
  Voltage Measurement3/LConn1 -- Voltage Measurement2/LConn2 -- Vc1/RConn1
  Vb1/RConn1 -- Voltage Measurement2/LConn1 -- Voltage Measurement1/LConn2
  Voltage Measurement8/LConn1 -- Voltage Measurement7/LConn2 -- Vb3/RConn1

== system eightenPulseRectifier/Controlled18PulseRectifier/Subsystem2 ==
  Three-Phase Transformer (Two Windings) : spsThreePhaseTransformerTwoWindingsLib/Three-Phase Transformer (Two Windings)  Winding1Connection=Yg  Winding2Connection=Yg  CoreType=Three single-phase transformers  SetSaturation=off  Hysteresis=off  DataFile='hysteresis'  SetInitialFlux=off  Measurements=None  UNITS=SI  NominalPower=[ 250e6 , 50 ]  Winding1=[253/sqrt(3) 0 0]  Winding2=[253/sqrt(3) 0 0]  Rm=1.0804e+06  Lm=2866  L0=0.5  Saturation=[0 0;0.66653 1910.3;277.72 2419.7]  InitialFluxes=[ 0.8 , -0.8 , 0.7 ]  BreakLoop=off  DiscreteSolver=Trapezoidal iterative  DataType=on  TransfoNumber=1
  Zigzag Phase-Shifting Transformer : spsZigzagPhaseShiftingTransformerLib/Zigzag Phase-Shifting Transformer  SecondaryConnection=Y  SetSaturation=off  SetInitialFlux=off  Measurements=None  UNITS=SI  NominalPower=[ 100e6 50]  PrimaryVoltage=200/sqrt(3)  SecondaryVoltage="[ 200/sqrt(3)  +20]"  Winding1=[0.000001 0.0000001]  Winding2=[0.000001 0.0000001]  Winding3=[0.000001 0.0000001]  RmLm=[622.01 1.6499]  Rm=622.01  Saturation=[0 0;17.569 28.988;7320.5 36.718]  InitialFluxes=[0 0 0]  BreakLoop=off  DiscreteSolver=Trapezoidal iterative  DataType=on
      settings: LibrarySourceBlock=|
      | sps_lib/Power Grid Elements/Zigzag
      | Phase-Shifting Transformer
  Zigzag Phase-Shifting Transformer1 : spsZigzagPhaseShiftingTransformerLib/Zigzag Phase-Shifting Transformer  SecondaryConnection=Y  SetSaturation=off  SetInitialFlux=off  Measurements=None  UNITS=SI  NominalPower=[ 100e6 50]  PrimaryVoltage=200/sqrt(3)  SecondaryVoltage="[ 200/sqrt(3)  -20]"  Winding1=[0.00001 0.000001]  Winding2=[0.00001 0.000001]  Winding3=[0.00001 0.000001]  RmLm=[622.01 1.6499]  Rm=622.01  Saturation=[0 0;17.569 28.988;7320.5 36.718]  InitialFluxes=[0 0 0]  BreakLoop=off  DiscreteSolver=Trapezoidal iterative  DataType=on
      settings: LibrarySourceBlock=|
      | sps_lib/Power Grid Elements/Zigzag
      | Phase-Shifting Transformer
  A : PMIOPort  Side=Left
  B : PMIOPort  Port=2  Side=Left
  C : PMIOPort  Port=3  Side=Left
  R1 : PMIOPort  Port=4  Side=Right
  S1 : PMIOPort  Port=5  Side=Right
  T1 : PMIOPort  Port=6  Side=Right
  R2 : PMIOPort  Port=7  Side=Right
  S2 : PMIOPort  Port=8  Side=Right
  T2 : PMIOPort  Port=9  Side=Right
  R3 : PMIOPort  Port=10  Side=Right
  S3 : PMIOPort  Port=11  Side=Right
  T3 : PMIOPort  Port=12  Side=Right
  connections:
  Three-Phase Transformer (Two Windings)/LConn3 -- C/RConn1 -- Zigzag Phase-Shifting Transformer/RConn3 -- Zigzag Phase-Shifting Transformer1/RConn3
  Three-Phase Transformer (Two Windings)/RConn1 -- R1/RConn1
  Three-Phase Transformer (Two Windings)/RConn2 -- S1/RConn1
  S2/RConn1 -- Zigzag Phase-Shifting Transformer/LConn2
  Three-Phase Transformer (Two Windings)/LConn2 -- B/RConn1 -- Zigzag Phase-Shifting Transformer/RConn2 -- Zigzag Phase-Shifting Transformer1/RConn2
  T2/RConn1 -- Zigzag Phase-Shifting Transformer/LConn3
  Zigzag Phase-Shifting Transformer1/LConn2 -- S3/RConn1
  Three-Phase Transformer (Two Windings)/RConn3 -- T1/RConn1
  Zigzag Phase-Shifting Transformer1/LConn3 -- T3/RConn1
  Three-Phase Transformer (Two Windings)/LConn1 -- A/RConn1 -- Zigzag Phase-Shifting Transformer/RConn1 -- Zigzag Phase-Shifting Transformer1/RConn1
  Zigzag Phase-Shifting Transformer/LConn6 -- Zigzag Phase-Shifting Transformer/LConn4 -- Zigzag Phase-Shifting Transformer/LConn5
  R2/RConn1 -- Zigzag Phase-Shifting Transformer/LConn1
  Zigzag Phase-Shifting Transformer1/LConn4 -- Zigzag Phase-Shifting Transformer1/LConn6 -- Zigzag Phase-Shifting Transformer1/LConn5
  Zigzag Phase-Shifting Transformer1/LConn1 -- R3/RConn1

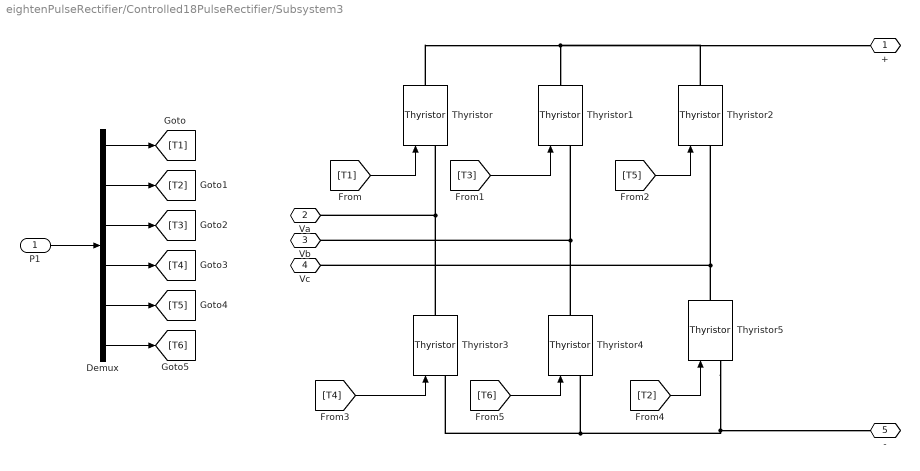
== system eightenPulseRectifier/Controlled18PulseRectifier/Subsystem3 ==
  P1 : Inport
  Demux : Demux  Outputs=6
  Thyristor{,1..5} (6 alike) : spsThyristorLib/Thyristor  Ron=0.001  Lon=0  Vf=0.8  IC=0  Rs=500  Cs=250e-9  Measurements=off
  + : PMIOPort  Side=Right
  Va : PMIOPort  Port=2  Side=Left
  Vb : PMIOPort  Port=3  Side=Left
  Vc : PMIOPort  Port=4  Side=Left
  - : PMIOPort  Port=5  Side=Right
  wires:
  Demux/1 -> [T1]
  Demux/2 -> [T2]
  Demux/3 -> [T3]
  Demux/4 -> [T4]
  Demux/5 -> [T5]
  Demux/6 -> [T6]
  P1/1 -> Demux/1
  [T1] -> Thyristor/1
  [T3] -> Thyristor1/1
  [T5] -> Thyristor2/1
  [T4] -> Thyristor3/1
  [T2] -> Thyristor5/1
  [T6] -> Thyristor4/1
  connections:
  Thyristor5/RConn1 -- Thyristor2/LConn1 -- Vc/RConn1
  Thyristor3/RConn1 -- Va/RConn1 -- Thyristor/LConn1
  Thyristor/RConn1 -- Thyristor1/RConn1 -- Thyristor2/RConn1 -- +/RConn1
  Thyristor5/LConn1 -- Thyristor4/LConn1 -- Thyristor3/LConn1 -- -/RConn1
  Thyristor4/RConn1 -- Thyristor1/LConn1 -- Vb/RConn1

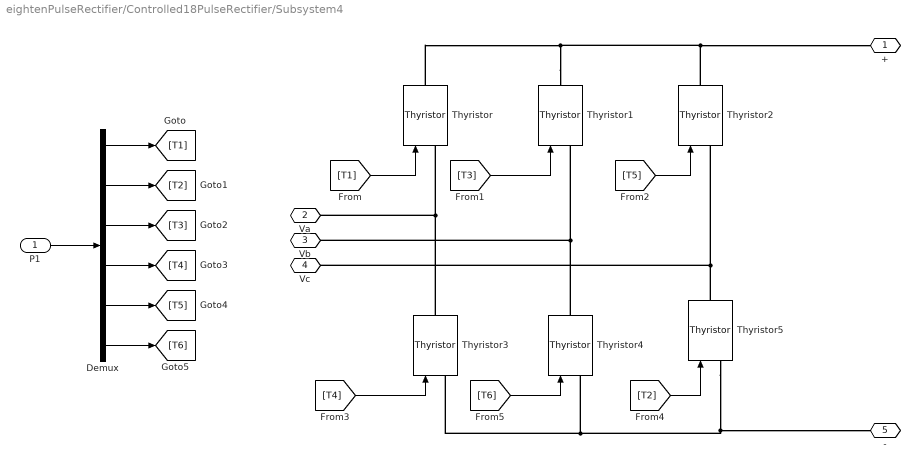
== system eightenPulseRectifier/Controlled18PulseRectifier/Subsystem4 ==
  P1 : Inport
  Demux : Demux  Outputs=6
  Thyristor{,1..5} (6 alike) : spsThyristorLib/Thyristor  Ron=0.001  Lon=0  Vf=0.8  IC=0  Rs=500  Cs=250e-9  Measurements=off
  + : PMIOPort  Side=Right
  Va : PMIOPort  Port=2  Side=Left
  Vb : PMIOPort  Port=3  Side=Left
  Vc : PMIOPort  Port=4  Side=Left
  - : PMIOPort  Port=5  Side=Right
  wires:
  [T6] -> Thyristor4/1
  [T2] -> Thyristor5/1
  [T4] -> Thyristor3/1
  [T5] -> Thyristor2/1
  [T3] -> Thyristor1/1
  [T1] -> Thyristor/1
  P1/1 -> Demux/1
  Demux/6 -> [T6]
  Demux/5 -> [T5]
  Demux/4 -> [T4]
  Demux/3 -> [T3]
  Demux/2 -> [T2]
  Demux/1 -> [T1]
  connections:
  Thyristor1/LConn1 -- Vb/RConn1 -- Thyristor4/RConn1
  -/RConn1 -- Thyristor5/LConn1 -- Thyristor3/LConn1 -- Thyristor4/LConn1
  Thyristor1/RConn1 -- Thyristor/RConn1 -- +/RConn1 -- Thyristor2/RConn1
  Va/RConn1 -- Thyristor/LConn1 -- Thyristor3/RConn1
  Thyristor2/LConn1 -- Vc/RConn1 -- Thyristor5/RConn1

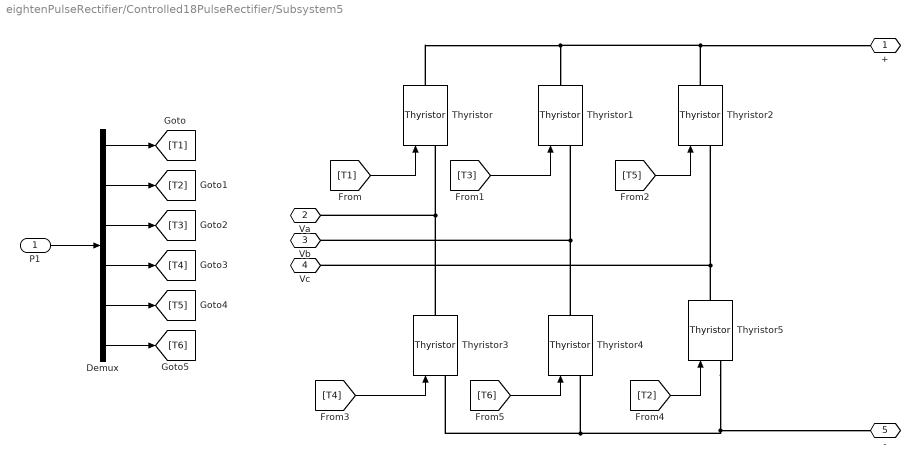
== system eightenPulseRectifier/Controlled18PulseRectifier/Subsystem5 ==
  P1 : Inport
  Demux : Demux  Outputs=6
  Thyristor{,1..5} (6 alike) : spsThyristorLib/Thyristor  Ron=0.001  Lon=0  Vf=0.8  IC=0  Rs=500  Cs=250e-9  Measurements=off
  + : PMIOPort  Side=Right
  Va : PMIOPort  Port=2  Side=Left
  Vb : PMIOPort  Port=3  Side=Left
  Vc : PMIOPort  Port=4  Side=Left
  - : PMIOPort  Port=5  Side=Right
  wires:
  Demux/1 -> [T1]
  Demux/2 -> [T2]
  Demux/3 -> [T3]
  Demux/4 -> [T4]
  Demux/5 -> [T5]
  Demux/6 -> [T6]
  P1/1 -> Demux/1
  [T1] -> Thyristor/1
  [T3] -> Thyristor1/1
  [T5] -> Thyristor2/1
  [T4] -> Thyristor3/1
  [T2] -> Thyristor5/1
  [T6] -> Thyristor4/1
  connections:
  Thyristor5/RConn1 -- Vc/RConn1 -- Thyristor2/LConn1
  Thyristor3/RConn1 -- Thyristor/LConn1 -- Va/RConn1
  Thyristor2/RConn1 -- +/RConn1 -- Thyristor/RConn1 -- Thyristor1/RConn1
  Thyristor4/LConn1 -- Thyristor3/LConn1 -- Thyristor5/LConn1 -- -/RConn1
  Thyristor4/RConn1 -- Vb/RConn1 -- Thyristor1/LConn1

== system eightenPulseRectifier/Controlled18PulseRectifier/Subsystem6 ==
  delayInDeg : Inport
  Freq : Inport  Port=2
  Add : Sum
  Add1 : Sum  Inputs=+-
  Add2 : Sum
  Constant1 : Constant  Value=360
  Constant4 : Constant  Value=20
  Constant6 : Constant  Value=20
  If : If  IfExpression=u1 < 0
  If Action Subsystem : Subsystem  TreatAsAtomicUnit=on
  If Action Subsystem1 : Subsystem  TreatAsAtomicUnit=on
  Merge : Merge
  Subsystem Reference : Subsystem  ReferencedSubsystem=DoublePulseFor6PulseRectifier
  Subsystem Reference1 : Subsystem  ReferencedSubsystem=DoublePulseFor6PulseRectifier
  Subsystem6 : Subsystem  ReferencedSubsystem=DoublePulseFor6PulseRectifier
  P1 : Outport
  P2 : Outport  Port=2
  P3 : Outport  Port=3
  wires:
  Freq/1 -> Subsystem Reference1/2, Subsystem Reference/2, Subsystem6/2
  Add1/1 -> If Action Subsystem1/1(In1), Add2/1, If/1
  delayInDeg/1 -> Add1/1, Add/1, Subsystem6/1
  Constant4/1 -> Add/2
  Constant6/1 -> Add1/2
  Add/1 -> Subsystem Reference/1
  Subsystem Reference1/1 -> P3/1
  Subsystem6/1 -> P1/1
  Subsystem Reference/1 -> P2/1
  If/1 -> If Action Subsystem/Action
  Add2/1 -> If Action Subsystem/1(In1)
  Constant1/1 -> Add2/2
  If/2 -> If Action Subsystem1/Action
  If Action Subsystem/1(Out1) -> Merge/1
  If Action Subsystem1/1(Out1) -> Merge/2
  Merge/1 -> Subsystem Reference1/1

== system eightenPulseRectifier/Controlled18PulseRectifierLPF/Subsystem ==
  freq : Inport
  Vll_RMS : Inport  Port=2
  Add : Sum
  Add1 : Sum
  Add2 : Sum
  Constant : Constant
  Gain : Gain  Gain=2*pi
  Gain1 : Gain  Gain=sqrt(2/3)
  Integrator : Integrator
  Product{,1..3} (4 alike) : Product
  Sin : Trigonometry
  Sin1 : Trigonometry
  Sin2 : Trigonometry
  phase : Constant  Value=0
  phase B : Constant  Value=-2*pi/3
  phase B1 : Constant  Value=2*pi/3
  PhA : Outport
  PhB : Outport  Port=2
  Phc : Outport  Port=3
  wires:
  Gain1/1 -> Product/2, Product3/2, Product1/2
  Gain/1 -> Product2/2  "2pit"
  Sin1/1 -> Product1/1
  Sin2/1 -> Product3/1
  Product1/1 -> PhB/1
  Product2/1 -> Add2/1, Add1/1, Add/1
  Integrator/1 -> Gain/1
  Constant/1 -> Integrator/1
  Vll_RMS/1 -> Gain1/1
  phase/1 -> Add/2
  phase B/1 -> Add1/2
  Add/1 -> Sin/1
  Add1/1 -> Sin1/1
  Add2/1 -> Sin2/1
  phase B1/1 -> Add2/2
  Product/1 -> PhA/1
  freq/1 -> Product2/1
  Product3/1 -> Phc/1
  Sin/1 -> Product/1

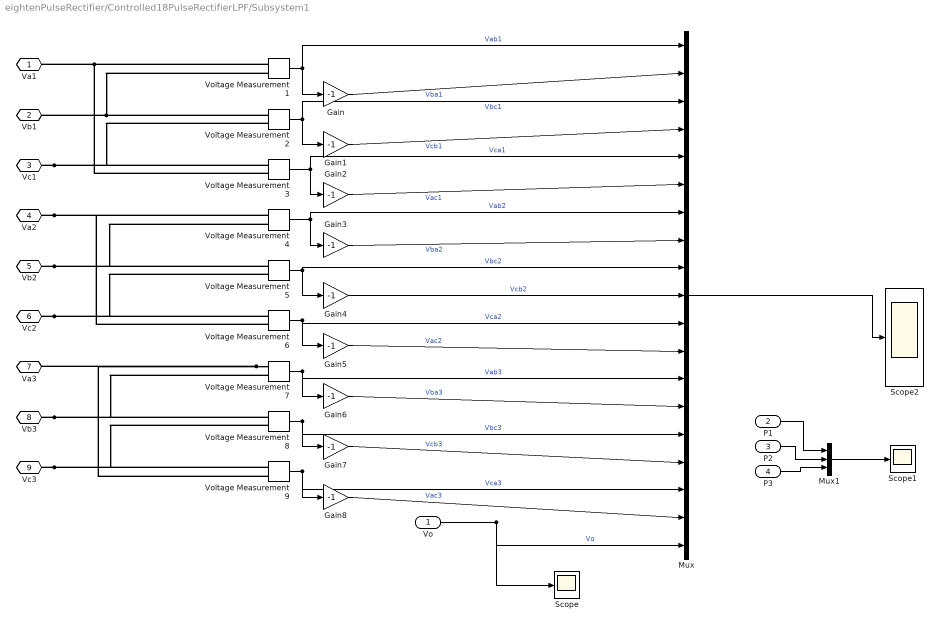
== system eightenPulseRectifier/Controlled18PulseRectifierLPF/Subsystem1 ==
  Vo : Inport
  P1 : Inport  Port=2
  P2 : Inport  Port=3
  P3 : Inport  Port=4
  Gain{,1..8} (9 alike) : Gain  Gain=-1
  Mux : Mux  Inputs=19
  Mux1 : Mux  Inputs=3
  Scope : Scope
  Scope1 : Scope
  Scope2 : Scope
  Voltage Measurement{1..9} (9 alike) : spsVoltageMeasurementLib/Voltage Measurement  PhasorSimulation=off  OutputType=Complex  PSBequivalent=0
  Va1 : PMIOPort  Side=Left
  Vb1 : PMIOPort  Port=2  Side=Left
  Vc1 : PMIOPort  Port=3  Side=Left
  Va2 : PMIOPort  Port=4  Side=Left
  Vb2 : PMIOPort  Port=5  Side=Left
  Vc2 : PMIOPort  Port=6  Side=Left
  Va3 : PMIOPort  Port=7  Side=Left
  Vb3 : PMIOPort  Port=8  Side=Left
  Vc3 : PMIOPort  Port=9  Side=Left
  wires:
  Mux1/1 -> Scope1/1
  P3/1 -> Mux1/3
  P2/1 -> Mux1/2
  P1/1 -> Mux1/1
  Mux/1 -> Scope2/1
  Vo/1 -> Mux/19, Scope/1  "Vo"
  Gain3/1 -> Mux/8  "Vba2"
  Gain6/1 -> Mux/14  "Vba3"
  Gain/1 -> Mux/2  "Vba1"
  Gain2/1 -> Mux/6  "Vac1"
  Gain4/1 -> Mux/10  "Vcb2"
  Voltage Measurement8/1 -> Gain7/1, Mux/15  "Vbc3"
  Voltage Measurement1/1 -> Mux/1, Gain/1  "Vab1"
  Voltage Measurement6/1 -> Mux/11, Gain5/1  "Vca2"
  Voltage Measurement7/1 -> Mux/13, Gain6/1  "Vab3"
  Gain5/1 -> Mux/12  "Vac2"
  Voltage Measurement9/1 -> Gain8/1, Mux/17  "Vca3"
  Gain7/1 -> Mux/16  "Vcb3"
  Gain8/1 -> Mux/18  "Vac3"
  Gain1/1 -> Mux/4  "Vcb1"
  Voltage Measurement3/1 -> Mux/5, Gain2/1  "Vca1"
  Voltage Measurement5/1 -> Mux/9, Gain4/1  "Vbc2"
  Voltage Measurement4/1 -> Mux/7, Gain3/1  "Vab2"
  Voltage Measurement2/1 -> Mux/3, Gain1/1  "Vbc1"
  connections:
  Vb3/RConn1 -- Voltage Measurement7/LConn2 -- Voltage Measurement8/LConn1
  Voltage Measurement1/LConn2 -- Voltage Measurement2/LConn1 -- Vb1/RConn1
  Vc1/RConn1 -- Voltage Measurement2/LConn2 -- Voltage Measurement3/LConn1
  Voltage Measurement7/LConn1 -- Va3/RConn1 -- Voltage Measurement9/LConn2
  Va2/RConn1 -- Voltage Measurement6/LConn2 -- Voltage Measurement4/LConn1
  Voltage Measurement3/LConn2 -- Voltage Measurement1/LConn1 -- Va1/RConn1
  Vb2/RConn1 -- Voltage Measurement4/LConn2 -- Voltage Measurement5/LConn1
  Vc3/RConn1 -- Voltage Measurement8/LConn2 -- Voltage Measurement9/LConn1
  Vc2/RConn1 -- Voltage Measurement5/LConn2 -- Voltage Measurement6/LConn1

== system eightenPulseRectifier/Controlled18PulseRectifierLPF/Subsystem2 ==
  Three-Phase Transformer (Two Windings) : spsThreePhaseTransformerTwoWindingsLib/Three-Phase Transformer (Two Windings)  Winding1Connection=Yg  Winding2Connection=Yg  CoreType=Three single-phase transformers  SetSaturation=off  Hysteresis=off  DataFile='hysteresis'  SetInitialFlux=off  Measurements=None  UNITS=SI  NominalPower=[ 250e6 , 50 ]  Winding1=[253/sqrt(3) 0 0]  Winding2=[253/sqrt(3) 0 0]  Rm=1.0804e+06  Lm=2866  L0=0.5  Saturation=[0 0;0.66653 1910.3;277.72 2419.7]  InitialFluxes=[ 0.8 , -0.8 , 0.7 ]  BreakLoop=off  DiscreteSolver=Trapezoidal iterative  DataType=on  TransfoNumber=1
  Zigzag Phase-Shifting Transformer : spsZigzagPhaseShiftingTransformerLib/Zigzag Phase-Shifting Transformer  SecondaryConnection=Y  SetSaturation=off  SetInitialFlux=off  Measurements=None  UNITS=SI  NominalPower=[ 100e6 50]  PrimaryVoltage=200/sqrt(3)  SecondaryVoltage="[ 200/sqrt(3)  +20]"  Winding1=[0.000001 0.0000001]  Winding2=[0.000001 0.0000001]  Winding3=[0.000001 0.0000001]  RmLm=[622.01 1.6499]  Rm=622.01  Saturation=[0 0;17.569 28.988;7320.5 36.718]  InitialFluxes=[0 0 0]  BreakLoop=off  DiscreteSolver=Trapezoidal iterative  DataType=on
      settings: LibrarySourceBlock=|
      | sps_lib/Power Grid Elements/Zigzag
      | Phase-Shifting Transformer
  Zigzag Phase-Shifting Transformer1 : spsZigzagPhaseShiftingTransformerLib/Zigzag Phase-Shifting Transformer  SecondaryConnection=Y  SetSaturation=off  SetInitialFlux=off  Measurements=None  UNITS=SI  NominalPower=[ 100e6 50]  PrimaryVoltage=200/sqrt(3)  SecondaryVoltage="[ 200/sqrt(3)  -20]"  Winding1=[0.00001 0.000001]  Winding2=[0.00001 0.000001]  Winding3=[0.00001 0.000001]  RmLm=[622.01 1.6499]  Rm=622.01  Saturation=[0 0;17.569 28.988;7320.5 36.718]  InitialFluxes=[0 0 0]  BreakLoop=off  DiscreteSolver=Trapezoidal iterative  DataType=on
      settings: LibrarySourceBlock=|
      | sps_lib/Power Grid Elements/Zigzag
      | Phase-Shifting Transformer
  A : PMIOPort  Side=Left
  B : PMIOPort  Port=2  Side=Left
  C : PMIOPort  Port=3  Side=Left
  R1 : PMIOPort  Port=4  Side=Right
  S1 : PMIOPort  Port=5  Side=Right
  T1 : PMIOPort  Port=6  Side=Right
  R2 : PMIOPort  Port=7  Side=Right
  S2 : PMIOPort  Port=8  Side=Right
  T2 : PMIOPort  Port=9  Side=Right
  R3 : PMIOPort  Port=10  Side=Right
  S3 : PMIOPort  Port=11  Side=Right
  T3 : PMIOPort  Port=12  Side=Right
  connections:
  Zigzag Phase-Shifting Transformer1/LConn1 -- R3/RConn1
  Zigzag Phase-Shifting Transformer1/LConn5 -- Zigzag Phase-Shifting Transformer1/LConn6 -- Zigzag Phase-Shifting Transformer1/LConn4
  R2/RConn1 -- Zigzag Phase-Shifting Transformer/LConn1
  Zigzag Phase-Shifting Transformer/LConn5 -- Zigzag Phase-Shifting Transformer/LConn4 -- Zigzag Phase-Shifting Transformer/LConn6
  Zigzag Phase-Shifting Transformer1/RConn1 -- Zigzag Phase-Shifting Transformer/RConn1 -- A/RConn1 -- Three-Phase Transformer (Two Windings)/LConn1
  Zigzag Phase-Shifting Transformer1/LConn3 -- T3/RConn1
  Three-Phase Transformer (Two Windings)/RConn3 -- T1/RConn1
  Zigzag Phase-Shifting Transformer1/LConn2 -- S3/RConn1
  T2/RConn1 -- Zigzag Phase-Shifting Transformer/LConn3
  Zigzag Phase-Shifting Transformer1/RConn2 -- Zigzag Phase-Shifting Transformer/RConn2 -- B/RConn1 -- Three-Phase Transformer (Two Windings)/LConn2
  S2/RConn1 -- Zigzag Phase-Shifting Transformer/LConn2
  Three-Phase Transformer (Two Windings)/RConn2 -- S1/RConn1
  Three-Phase Transformer (Two Windings)/RConn1 -- R1/RConn1
  Zigzag Phase-Shifting Transformer1/RConn3 -- Zigzag Phase-Shifting Transformer/RConn3 -- C/RConn1 -- Three-Phase Transformer (Two Windings)/LConn3

== system eightenPulseRectifier/Controlled18PulseRectifierLPF/Subsystem3 ==
  P1 : Inport
  Demux : Demux  Outputs=6
  Thyristor{,1..5} (6 alike) : spsThyristorLib/Thyristor  Ron=0.001  Lon=0  Vf=0.8  IC=0  Rs=500  Cs=250e-9  Measurements=off
  + : PMIOPort  Side=Right
  Va : PMIOPort  Port=2  Side=Left
  Vb : PMIOPort  Port=3  Side=Left
  Vc : PMIOPort  Port=4  Side=Left
  - : PMIOPort  Port=5  Side=Right
  wires:
  [T6] -> Thyristor4/1
  [T2] -> Thyristor5/1
  [T4] -> Thyristor3/1
  [T5] -> Thyristor2/1
  [T3] -> Thyristor1/1
  [T1] -> Thyristor/1
  P1/1 -> Demux/1
  Demux/6 -> [T6]
  Demux/5 -> [T5]
  Demux/4 -> [T4]
  Demux/3 -> [T3]
  Demux/2 -> [T2]
  Demux/1 -> [T1]
  connections:
  Vb/RConn1 -- Thyristor1/LConn1 -- Thyristor4/RConn1
  -/RConn1 -- Thyristor3/LConn1 -- Thyristor4/LConn1 -- Thyristor5/LConn1
  +/RConn1 -- Thyristor2/RConn1 -- Thyristor1/RConn1 -- Thyristor/RConn1
  Thyristor/LConn1 -- Va/RConn1 -- Thyristor3/RConn1
  Vc/RConn1 -- Thyristor2/LConn1 -- Thyristor5/RConn1

== system eightenPulseRectifier/Controlled18PulseRectifierLPF/Subsystem4 ==
  P1 : Inport
  Demux : Demux  Outputs=6
  Thyristor{,1..5} (6 alike) : spsThyristorLib/Thyristor  Ron=0.001  Lon=0  Vf=0.8  IC=0  Rs=500  Cs=250e-9  Measurements=off
  + : PMIOPort  Side=Right
  Va : PMIOPort  Port=2  Side=Left
  Vb : PMIOPort  Port=3  Side=Left
  Vc : PMIOPort  Port=4  Side=Left
  - : PMIOPort  Port=5  Side=Right
  wires:
  Demux/1 -> [T1]
  Demux/2 -> [T2]
  Demux/3 -> [T3]
  Demux/4 -> [T4]
  Demux/5 -> [T5]
  Demux/6 -> [T6]
  P1/1 -> Demux/1
  [T1] -> Thyristor/1
  [T3] -> Thyristor1/1
  [T5] -> Thyristor2/1
  [T4] -> Thyristor3/1
  [T2] -> Thyristor5/1
  [T6] -> Thyristor4/1
  connections:
  Thyristor5/RConn1 -- Vc/RConn1 -- Thyristor2/LConn1
  Thyristor3/RConn1 -- Thyristor/LConn1 -- Va/RConn1
  Thyristor2/RConn1 -- +/RConn1 -- Thyristor/RConn1 -- Thyristor1/RConn1
  Thyristor4/LConn1 -- Thyristor3/LConn1 -- Thyristor5/LConn1 -- -/RConn1
  Thyristor4/RConn1 -- Vb/RConn1 -- Thyristor1/LConn1

== system eightenPulseRectifier/Controlled18PulseRectifierLPF/Subsystem5 ==
  P1 : Inport
  Demux : Demux  Outputs=6
  Thyristor{,1..5} (6 alike) : spsThyristorLib/Thyristor  Ron=0.001  Lon=0  Vf=0.8  IC=0  Rs=500  Cs=250e-9  Measurements=off
  + : PMIOPort  Side=Right
  Va : PMIOPort  Port=2  Side=Left
  Vb : PMIOPort  Port=3  Side=Left
  Vc : PMIOPort  Port=4  Side=Left
  - : PMIOPort  Port=5  Side=Right
  wires:
  [T6] -> Thyristor4/1
  [T2] -> Thyristor5/1
  [T4] -> Thyristor3/1
  [T5] -> Thyristor2/1
  [T3] -> Thyristor1/1
  [T1] -> Thyristor/1
  P1/1 -> Demux/1
  Demux/6 -> [T6]
  Demux/5 -> [T5]
  Demux/4 -> [T4]
  Demux/3 -> [T3]
  Demux/2 -> [T2]
  Demux/1 -> [T1]
  connections:
  Thyristor1/LConn1 -- Vb/RConn1 -- Thyristor4/RConn1
  -/RConn1 -- Thyristor5/LConn1 -- Thyristor3/LConn1 -- Thyristor4/LConn1
  Thyristor1/RConn1 -- Thyristor/RConn1 -- +/RConn1 -- Thyristor2/RConn1
  Va/RConn1 -- Thyristor/LConn1 -- Thyristor3/RConn1
  Thyristor2/LConn1 -- Vc/RConn1 -- Thyristor5/RConn1

== system eightenPulseRectifier/Controlled18PulseRectifierLPF/Subsystem6 ==
  delayInDeg : Inport
  Freq : Inport  Port=2
  Add : Sum
  Add1 : Sum  Inputs=+-
  Add2 : Sum
  Constant1 : Constant  Value=360
  Constant4 : Constant  Value=20
  Constant6 : Constant  Value=20
  If : If  IfExpression=u1 < 0
  If Action Subsystem : Subsystem  TreatAsAtomicUnit=on
  If Action Subsystem1 : Subsystem  TreatAsAtomicUnit=on
  Merge : Merge
  Subsystem Reference : Subsystem  ReferencedSubsystem=DoublePulseFor6PulseRectifier
  Subsystem Reference1 : Subsystem  ReferencedSubsystem=DoublePulseFor6PulseRectifier
  Subsystem6 : Subsystem  ReferencedSubsystem=DoublePulseFor6PulseRectifier
  P1 : Outport
  P2 : Outport  Port=2
  P3 : Outport  Port=3
  wires:
  Merge/1 -> Subsystem Reference1/1
  If Action Subsystem1/1(Out1) -> Merge/2
  If Action Subsystem/1(Out1) -> Merge/1
  If/2 -> If Action Subsystem1/Action
  Constant1/1 -> Add2/2
  Add2/1 -> If Action Subsystem/1(In1)
  If/1 -> If Action Subsystem/Action
  Subsystem Reference/1 -> P2/1
  Subsystem6/1 -> P1/1
  Subsystem Reference1/1 -> P3/1
  Add/1 -> Subsystem Reference/1
  Constant6/1 -> Add1/2
  Constant4/1 -> Add/2
  delayInDeg/1 -> Subsystem6/1, Add/1, Add1/1
  Add1/1 -> If/1, Add2/1, If Action Subsystem1/1(In1)
  Freq/1 -> Subsystem6/2, Subsystem Reference/2, Subsystem Reference1/2
